simulink model "untitled100"  (R2013a)
settings: Solver=ode45  StartTime=0.0  StopTime=10  RelTol=1e-3
values from neighbouring files (symbols this model uses):
  a = [0,0,1,0;0,0,0,1;0,-289.47,-3.98,0;0,103.05,-1.97,0]    [Untitled10.m]
  b = [0;0;9.057;5.655]    [Untitled10.m]
  c = [1,0,0,0;0,1,0,0;0,0,1,0;0,0,0,1]    [Untitled10.m]
  d = [0;0;0;0]    [Untitled10.m]
  g = 9.8    [Untitled10.m]
  jp = 2.26e-3    (= 0.00226)    [Untitled10.m]
  jw = 2.312e-5    (= 2.312e-05)    [Untitled10.m]
  Ke = 0.44    [Untitled10.m]
  Kt = 0.47    [Untitled10.m]
  l = 0.04    [Untitled10.m]
  mp = 0.57    [Untitled10.m]
  mw = 0.04    [Untitled10.m]
  n = 1/20    (= 0.05)    [Untitled10.m]
  r = 0.034    [Untitled10.m]
  Ra = 9.5    [Untitled10.m]
undefined symbols (not defined in the file or in its folder): fdesignblkfcn, gcbh, jb, psi, psidot, tethadot, thetadot
libraries: simulink x2
settings Model: Creator=user  LastModifiedBy=user

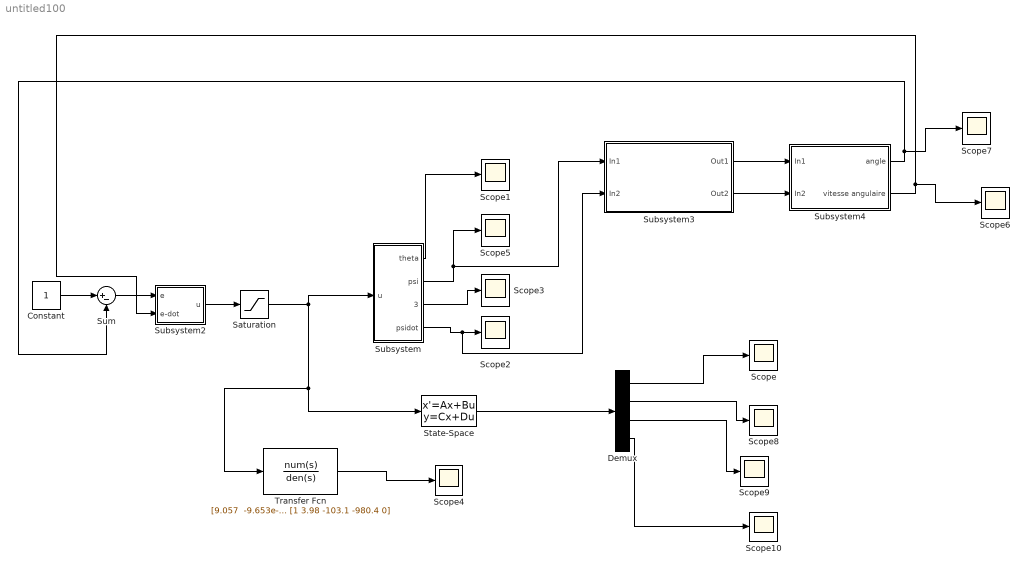
== system untitled100 ==
  Constant : Constant
  Demux : Demux
  Saturation : Saturate
  Scope{,1..10} (11 alike) : Scope
      Scope1 settings: SaveName=ScopeData5
      Scope10 settings: SaveName=ScopeData3
      Scope2 settings: SaveName=ScopeData6
      Scope3 settings: SaveName=ScopeData7
      Scope4 settings: SaveName=ScopeData4
      Scope5 settings: SaveName=ScopeData8
      Scope6 settings: SaveName=ScopeData9
      Scope7 settings: SaveName=ScopeData10
      Scope9 settings: SaveName=ScopeData2
  State-Space : StateSpace  A=a  B=b  C=c  D=d
  Subsystem : Subsystem
  Subsystem2 : Subsystem
  Subsystem3 : Subsystem
  Subsystem4 : Subsystem
  Sum : Sum  Inputs=|+-
  Transfer Fcn : TransferFcn  Numerator="[9.057  -9.653e-14 -2570]"  Denominator=[1 3.98 -103.1 -980.4 0]
  wires:
  Constant/1 -> Sum/1
  Sum/1 -> Subsystem2/1(e)
  Subsystem2/1(u) -> Saturation/1
  Subsystem/1(theta) -> Scope1/1
  Subsystem/4(psidot) -> Subsystem3/2(In2), Scope2/1
  Subsystem/2(psi) -> Scope5/1, Subsystem3/1(In1)
  Subsystem/3(thetadot) -> Scope3/1
  Subsystem3/1(Out1) -> Subsystem4/1(In1)
  Subsystem3/2(Out2) -> Subsystem4/2(In2)
  Subsystem4/1("angle ") -> Sum/2, Scope7/1
  Subsystem4/2(vitesse angulaire) -> Subsystem2/2(e-dot), Scope6/1
  State-Space/1 -> Demux/1
  Demux/1 -> Scope/1
  Demux/2 -> Scope8/1
  Demux/3 -> Scope9/1
  Demux/4 -> Scope10/1
  Saturation/1 -> Transfer Fcn/1, State-Space/1, Subsystem/1(u)
  Transfer Fcn/1 -> Scope4/1

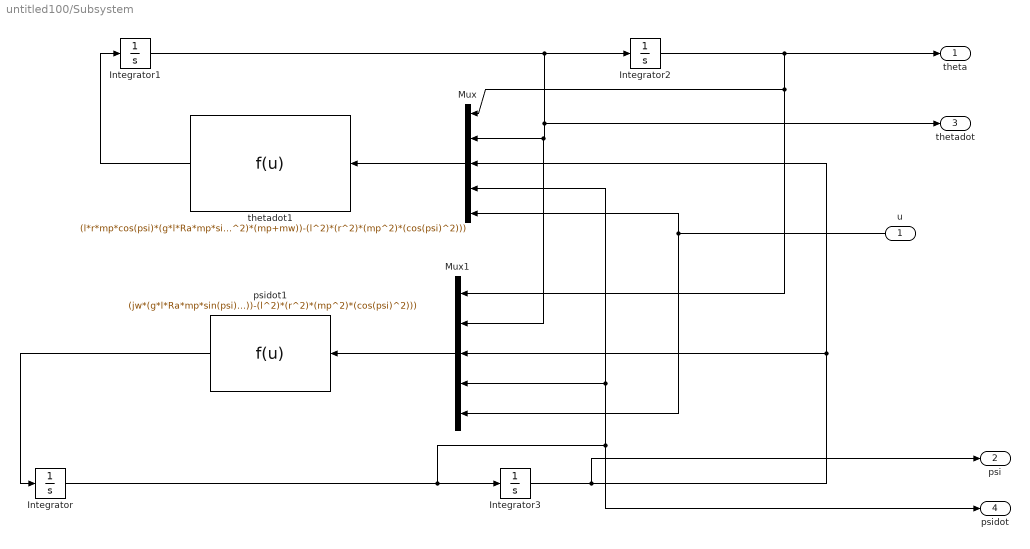
== system untitled100/Subsystem ==
  u : Inport
  Integrator{,1..3} (4 alike) : Integrator
  Mux : Mux  Inputs=5
  Mux1 : Mux  Inputs=5
  psidot1 : Fcn  Expr=(jw*(g*l*Ra*mp*sin(psi)+2*n*Kt*(u-Ke*thetadot))+r*(l*r*Ra*mp*sin(psi)*(mp*(g-l*((psidot)^2)*cos(psi))+g*mw)+2*n*Kt*(u-Ke*tethadot)*(mp*(l*cos(psi)+r)+r*mw)))/Ra*(jp*(jw+(r^2)*(mp+mw))-(l^2)*(r^2)*(mp^2)*(cos(psi)^2)))
  thetadot1 : Fcn  Expr=(l*r*mp*cos(psi)*(g*l*Ra*mp*sin(psi))+2*n*Kt*(u-Ke*thetadot))+jp*(2*n*Kt(u-Ke*thetadot)-l*r*Ra*mp*(psidot^2)*sin(psi))/(Ra*(jb*(jw+(r^2)*(mp+mw))-(l^2)*(r^2)*(mp^2)*(cos(psi)^2)))
  theta : Outport
  psi : Outport  Port=2
  thetadot : Outport  Port=3
  psidot : Outport  Port=4
  wires:
  Mux/1 -> thetadot1/1
  thetadot1/1 -> Integrator1/1
  Integrator1/1 -> Mux1/2, Mux/2, thetadot/1, Integrator2/1
  Integrator2/1 -> Mux1/1, Mux/1, theta/1
  Mux1/1 -> psidot1/1
  Integrator/1 -> Mux/4, Mux1/4, psidot/1, Integrator3/1
  Integrator3/1 -> Mux/3, Mux1/3, psi/1
  u/1 -> Mux1/5, Mux/5
  psidot1/1 -> Integrator/1

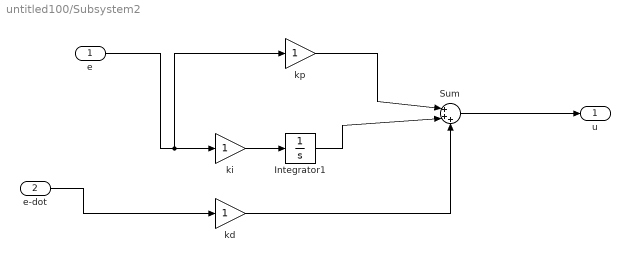
== system untitled100/Subsystem2 ==
  e : Inport
  e-dot : Inport  Port=2
  Integrator1 : Integrator
  Sum : Sum  Inputs=|+++
  kd : Gain
  ki : Gain
  kp : Gain
  u : Outport
  wires:
  kp/1 -> Sum/1
  ki/1 -> Integrator1/1
  Sum/1 -> u/1
  kd/1 -> Sum/3
  Integrator1/1 -> Sum/2
  e/1 -> kp/1, ki/1
  e-dot/1 -> kd/1

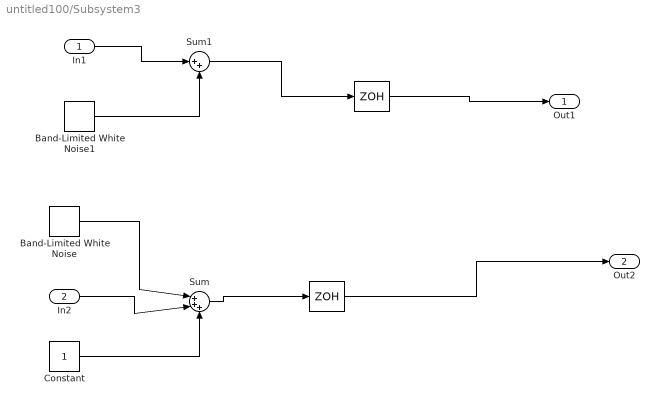
== system untitled100/Subsystem3 ==
  In1 : Inport
  In2 : Inport  Port=2
  " " : ZeroOrderHold
  " " : ZeroOrderHold
  Band-Limited White Noise : simulink/Sources/Band-Limited White Noise  Cov=[0.1]  Ts=0.1  seed=[23341]
  Band-Limited White Noise1 : simulink/Sources/Band-Limited White Noise  Cov=[0.1]  Ts=0.1  seed=[23341]
  Constant : Constant
  Sum : Sum  Inputs=|+++
  Sum1 : Sum  Inputs=|++
  Out1 : Outport
  Out2 : Outport  Port=2
  wires:
  In1/1 -> Sum1/1
  Band-Limited White Noise1/1 -> Sum1/2
  Band-Limited White Noise/1 -> Sum/1
  In2/1 -> Sum/2
  Constant/1 -> Sum/3
  Sum/1 -> " "/1
  Sum1/1 -> " "/1
  " "/1 -> Out1/1
  " "/1 -> Out2/1

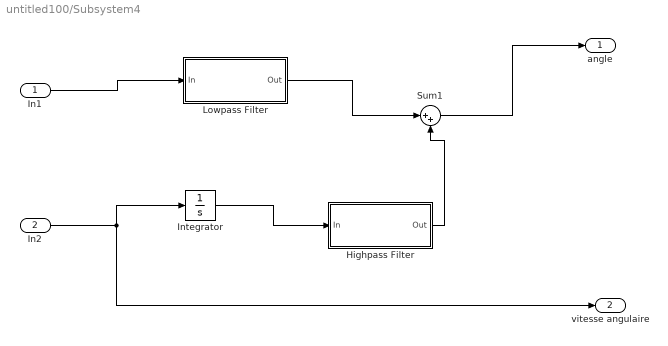
== system untitled100/Subsystem4 ==
  In1 : Inport
  In2 : Inport  Port=2
  Highpass Filter : Subsystem  DialogController=fdesignblkfcn  InitFcn=fdesignblkfcn(gcbh, {'InitFcn'});  mask(Highpass Filter){}
      mask help: Design a highpass filter
      settings: CopyFcn=fdesignblkfcn(gcbh, {'CopyFcn'});
      mask Help: helpview(mapfilelocation('dsp'), 'dsphighpassfilter');
      mask Display: disp('Highpass')
  Integrator : Integrator
  Lowpass Filter : Subsystem  DialogController=fdesignblkfcn  InitFcn=fdesignblkfcn(gcbh, {'InitFcn'});  mask(Lowpass Filter){}
      mask help: Design a lowpass filter
      settings: CopyFcn=fdesignblkfcn(gcbh, {'CopyFcn'});
      mask Help: helpview(mapfilelocation('dsp'), 'dsplowpassfilter');
      mask Display: disp('Lowpass')
  Sum1 : Sum  Inputs=|++
  "angle " : Outport
  vitesse angulaire : Outport  Port=2
  wires:
  Integrator/1 -> Highpass Filter/1(In)
  In2/1 -> vitesse angulaire/1, Integrator/1
  Highpass Filter/1(Out) -> Sum1/2
  Lowpass Filter/1(Out) -> Sum1/1
  In1/1 -> Lowpass Filter/1(In)
  Sum1/1 -> "angle "/1

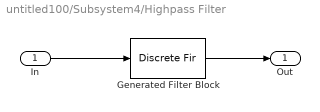
== system untitled100/Subsystem4/Highpass Filter ==
  In : Inport
  Generated Filter Block : DiscreteFir  Tag=BlockMethodSubSystem  Coefficients=[-0.001713682665110306 0.0083143784480805769 -0.012717355233486931 0.0055609517902503753 0.0073397102425536197 -0.006531049050179258 -0.0076900499697794954 0.0090269831680985079 0.0088388618995090904 -0.012960741353766195 -0.010074958667252783 0.018520174010008873 0.011233354613588929 -0.026375248383613631 -0.012270782185765867 0.038180976692389727 0.013130425918293593 -0.058293359325192265 -0.013768295948648092 0.102813257992074 0.014167876773854067 -0.31720255241603534 0.48569804617051759 -0.31720255241603534 0.014167876773854067 0.102813257992074 -0.013768295948648092 -0.058293359325192265 0.013130425918293593 0.038180976692389727 -0.012270782185765867 -0.026375248383613631 0.011233354613588929 0.018520174010008873 -0.010074958667252783 -0.012960741353766195 0.0088388618995090904 0.0090269831680985079 -0.0076900499697794954 -0.006531049050179258 0.0073397102425536197 0.0055609517902503753 -0.012717355233486931 0.0083143784480805769 -0.001713682665110306]  InputProcessing=Columns as channels (frame based)
  Out : Outport
  wires:
  Generated Filter Block/1 -> Out/1
  In/1 -> Generated Filter Block/1

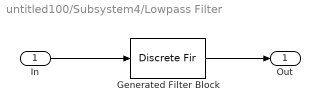
== system untitled100/Subsystem4/Lowpass Filter ==
  In : Inport
  Generated Filter Block : DiscreteFir  Tag=BlockMethodSubSystem  Coefficients=[-0.0024228738523269142 -0.002083244982079274 0.0067703446401187091 0.016731945423489058 0.011117076081077608 -0.0062311454141445394 -0.008401617186026911 0.0092567976151380175 0.012982883808855752 -0.010121234703278968 -0.018273518733782485 0.011431962071777957 0.02617588858040763 -0.012489027835322923 -0.037996623145463579 0.013388945199366963 0.058155465814729891 -0.014048043515808939 -0.10272466857882172 0.014462275771238358 0.31716649721769491 0.48538764678732504 0.31716649721769491 0.014462275771238358 -0.10272466857882172 -0.014048043515808939 0.058155465814729891 0.013388945199366963 -0.037996623145463579 -0.012489027835322923 0.02617588858040763 0.011431962071777957 -0.018273518733782485 -0.010121234703278968 0.012982883808855752 0.0092567976151380175 -0.008401617186026911 -0.0062311454141445394 0.011117076081077608 0.016731945423489058 0.0067703446401187091 -0.002083244982079274 -0.0024228738523269142]  InputProcessing=Columns as channels (frame based)
  Out : Outport
  wires:
  In/1 -> Generated Filter Block/1
  Generated Filter Block/1 -> Out/1
